simulink model "WheelSlipKinematics"  (R2026b)
settings: Solver=ode45  StopTime=1
undefined symbols (not defined in the file): Tire
settings Model: DataDictionary=VehicleData.sldd  Creator=Xu Dingyi  LastModifiedBy=29358

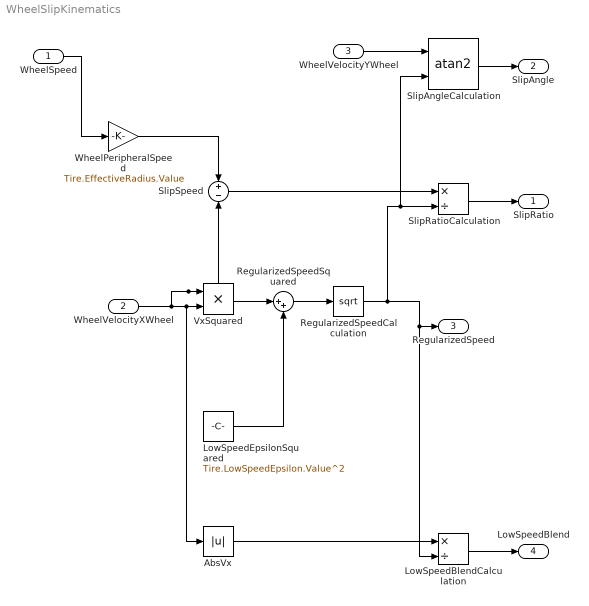
== system WheelSlipKinematics ==
  WheelSpeed : Inport  OutDataTypeStr=double  PortDimensions=[4 1]
  WheelVelocityXWheel : Inport  Port=2  OutDataTypeStr=double  PortDimensions=[4 1]
  WheelVelocityYWheel : Inport  Port=3  OutDataTypeStr=double  PortDimensions=[4 1]
  AbsVx : Abs
  LowSpeedBlendCalculation : Product  Inputs=*/
  LowSpeedEpsilonSquared : Constant  Value=Tire.LowSpeedEpsilon.Value^2  OutDataTypeStr=double
  RegularizedSpeedCalculation : Sqrt
  RegularizedSpeedSquared : Sum  Inputs=|++
  SlipAngleCalculation : Trigonometry  Operator=atan2
  SlipRatioCalculation : Product  Inputs=*/
  SlipSpeed : Sum  Inputs=+-
  VxSquared : Product  Inputs=**
  WheelPeripheralSpeed : Gain  Gain=Tire.EffectiveRadius.Value
  SlipRatio : Outport
  SlipAngle : Outport  Port=2
  RegularizedSpeed : Outport  Port=3
  LowSpeedBlend : Outport  Port=4
  wires:
  AbsVx/1 -> LowSpeedBlendCalculation/1
  WheelVelocityYWheel/1 -> SlipAngleCalculation/1
  RegularizedSpeedCalculation/1 -> LowSpeedBlendCalculation/2, RegularizedSpeed/1, SlipRatioCalculation/2, SlipAngleCalculation/2
  SlipSpeed/1 -> SlipRatioCalculation/1
  WheelPeripheralSpeed/1 -> SlipSpeed/1
  RegularizedSpeedSquared/1 -> RegularizedSpeedCalculation/1
  LowSpeedEpsilonSquared/1 -> RegularizedSpeedSquared/2
  VxSquared/1 -> RegularizedSpeedSquared/1
  WheelVelocityXWheel/1 -> VxSquared/2, AbsVx/1, VxSquared/1, SlipSpeed/2
  WheelSpeed/1 -> WheelPeripheralSpeed/1
  SlipRatioCalculation/1 -> SlipRatio/1
  SlipAngleCalculation/1 -> SlipAngle/1
  LowSpeedBlendCalculation/1 -> LowSpeedBlend/1
